simulink model "Demo_M1V4_UNO"  (R2015a)
settings: Solver=FixedStepDiscrete  StartTime=0.0  StopTime=inf  FixedStep=.03  RelTol=1e-3
libraries: RASPlib x3, arduinolib x3, MinSegLibrary_M1V4 x2
settings Model: ExtModeTrigDuration=2  Creator=Alec  LastModifiedBy=hurstj
settings OptimizationCC: ExpressionDepthLimit=2147483647  OptimizeModelRefInitCode=on  LifeSpan=1
settings DebuggingCC: UnderspecifiedInitializationDetection=Classic  MergeDetectMultiDrivingBlocksExec=none  StateNameClashWarn=warning
settings HardwareCC: ProdBitPerInt=16  ProdBitPerPointer=8  ProdIntDivRoundTo=Zero  ProdEndianess=LittleEndian  ProdWordSize=8  ProdHWDeviceType=Atmel->AVR
settings RTWCC: SystemTargetFile=realtime.tlc  GenerateMakefile=off  TemplateMakefile=realtime.tmf  Description=Real-Time Toolbox  RTWVerbose=off
settings CodeAppCC: CustomSymbolStrType=$N$R$M  InternalIdentifier=Classic
settings ERTTargetCC: CombineOutputUpdateFcns=off  ExtModeTransport=3  ExtModeMexArgs=0 1 9600  ERTSrcFileBannerTemplate=realtime_code_template.cgt  ERTHdrFileBannerTemplate=realtime_code_template.cgt  ERTDataSrcFileTemplate=realtime_code_template.cgt  ERTDataHdrFileTemplate=realtime_code_template.cgt  ERTCustomFileTemplate=realtime_file_process.tlc

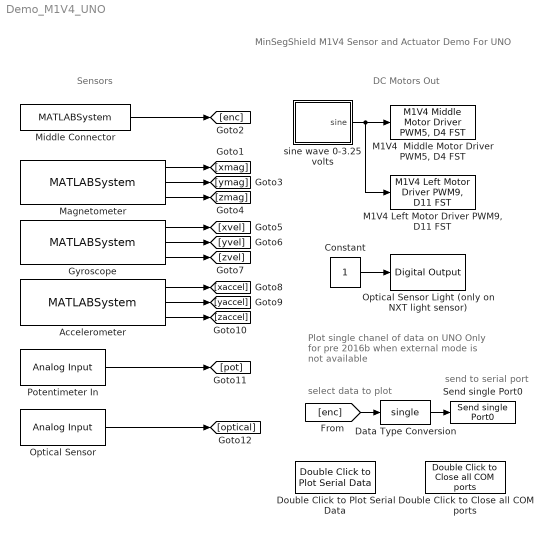
== system Demo_M1V4_UNO ==
  note: send to serial port
  note: select data to plot
  note: Plot single chanel of data on UNO
      | Only for pre 2016b when external
      | mode is not available
  note: DC Motors Out
  note: Sensors
  note: MinSegShield M1V4 Sensor and Actuator Demo
      | For UNO
  Accelerometer : MATLABSystem  System=soMPU6050Accel  SimulateUsing=Code generation
      mask Type: soMPU6050Accel
      mask Display:
      | disp('soMPU6050Accel');
      | port_label('output',1,'xaccel');
      | port_label('output',2,'yaccel');
      | port_label('output',3,'zaccel');
  Constant : Constant
  Data Type Conversion : DataTypeConversion  OutDataTypeStr=single
  Double Click to Close all COM ports : RASPlib/Double Click to Close all COM ports
  Double Click to Plot Serial Data : RASPlib/Double Click to Plot Serial Data  COMport=4  BaudRate=115200  NumSamples=500  DataType=uint8  Ncx=1
  Gyroscope : MATLABSystem  System=soMPU6050Gyro  DLPFmode=0
      mask Type: soMPU6050Gyro
      mask Display:
      | disp('soMPU6050Gyro');
      | port_label('output',1,'xvel');
      | port_label('output',2,'yvel');
      | port_label('output',3,'zvel');
  "M1V4  Middle Motor Driver PWM5, D4 FST" : MinSegLibrary_M1V4/M1V4  Middle Motor Driver PWM5, D4 FST  Vsupply=3.25
  "M1V4 Left Motor Driver PWM9, D11 FST" : MinSegLibrary_M1V4/M1V4 Left Motor Driver PWM9, D11 FST  Vsupply=3.25
  Magnetometer : MATLABSystem  System=soHMC5883L  SimulateUsing=Code generation
      mask Type: soHMC5883L
      mask Display:
      | disp('soHMC5883L');
      | port_label('output',1,'xmag');
      | port_label('output',2,'ymag');
      | port_label('output',3,'zmag');
  Middle Connector : MATLABSystem  System=Encoder_arduino_uno_nano  Encoder=0  PinA=2  PinB=3
      mask Type: Encoder_arduino_uno_nano
      mask Display:
      | disp('soEncoder');
      | port_label('output',1,'y');
  Optical Sensor : arduinolib/Analog Input  pinNumber=1  sampleTime=-1  blockPlatform=arduino
  Optical Sensor Light (only on NXT light sensor) : arduinolib/Digital Output  pinNumber=12  blockPlatform=arduino
  Potentimeter In : arduinolib/Analog Input  pinNumber=0  sampleTime=-1  blockPlatform=arduino
  Send single Port0 : RASPlib/Send single Port0
  sine wave 0-3.25 volts : Subsystem
  wires:
  sine wave 0-3.25 volts/1(sine) -> "M1V4 Left Motor Driver PWM9, D11 FST"/1, "M1V4  Middle Motor Driver PWM5, D4 FST"/1
  Potentimeter In/1 -> [pot]
  Optical Sensor/1 -> [optical]
  Constant/1 -> Optical Sensor Light (only on NXT light sensor)/1
  Middle Connector/1 -> [enc]
  Magnetometer/1 -> [xmag]
  Magnetometer/2 -> [ymag]
  Magnetometer/3 -> [zmag]
  Gyroscope/1 -> [xvel]
  Gyroscope/2 -> [yvel]
  Gyroscope/3 -> [zvel]
  Accelerometer/1 -> [xaccel]
  Accelerometer/2 -> [yaccel]
  Accelerometer/3 -> [zaccel]
  [enc] -> Data Type Conversion/1
  Data Type Conversion/1 -> Send single Port0/1

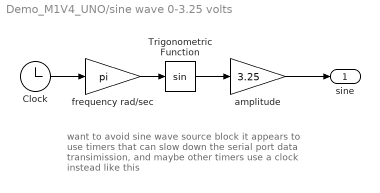
== system Demo_M1V4_UNO/sine wave 0-3.25 volts ==
  note: want to avoid sine wave source block
      | it appears to use timers that can slow down the
      | serial port data transimission, and maybe
      | other timers
      |
      | use a clock instead like this
  Clock : Clock
  Trigonometric Function : Trigonometry
  amplitude : Gain  Gain=3.25
  frequency rad/sec : Gain  Gain=pi
  sine : Outport
  wires:
  Clock/1 -> frequency rad/sec/1
  Trigonometric Function/1 -> amplitude/1
  frequency rad/sec/1 -> Trigonometric Function/1
  amplitude/1 -> sine/1
